simulink subsystem "TIME"  (R2025b)
settings: Solver=VariableStepAuto  StartTime=0.0  StopTime=10.0  RelTol=1e-3
model mask{initPosixTime=0, refPosixTime=0}
  mask prompts: initPosixTime "Initial time (UTC, Posix format)"; refPosixTime "Reference time (UTC, Posix format)"
settings Model: Creator=antoniohernandez-rodiciomateos  LastModifiedBy=antoniohernandez-rodiciomateos

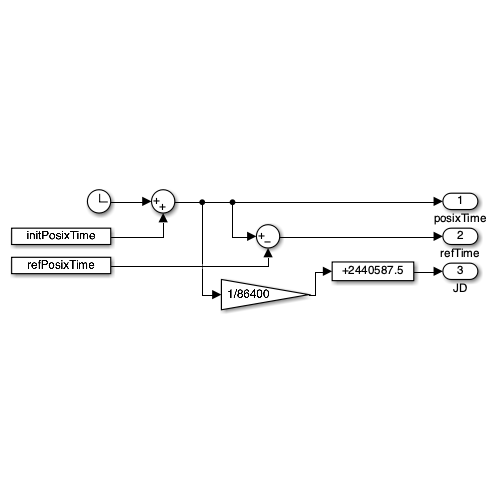
[thumbnail: Simulink's stored preview of the top-level diagram]
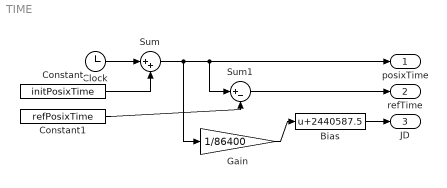
== system TIME ==
  Bias : Bias  Bias=2440587.5  SaturateOnIntegerOverflow=off
  Clock : Clock
  Constant : Constant  Value=initPosixTime
  Constant1 : Constant  Value=refPosixTime
  Gain : Gain  Gain=1/86400
  Sum : Sum  Inputs=|++
  Sum1 : Sum  Inputs=|+-
  posixTime : Outport
  refTime : Outport  Port=2
  JD : Outport  Port=3
  wires:
  Clock/1 -> Sum/1
  Constant/1 -> Sum/2
  Sum/1 -> Gain/1, Sum1/1, posixTime/1
  Sum1/1 -> refTime/1
  Constant1/1 -> Sum1/2
  Gain/1 -> Bias/1
  Bias/1 -> JD/1
